simulink model "parcheggioAssistito_Simu"  (R2023a)
settings: Solver=VariableStepAuto  StartTime=0.0  StopTime=30.0  RelTol=1e-3
undefined symbols (not defined in the file or in its folder): ZigBee
libraries: truetime x12, fuzblock x1
settings Model: Creator=elisa  LastModifiedBy=elisa

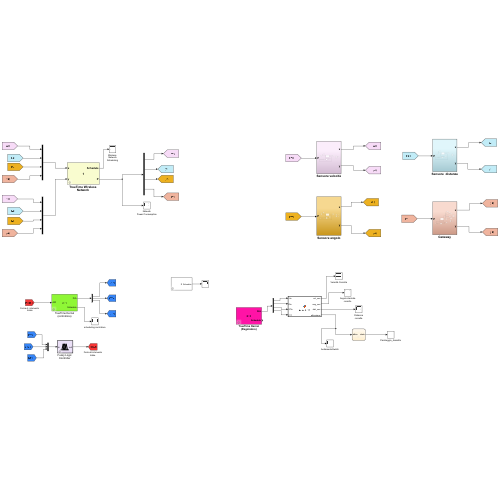
[thumbnail: Simulink's stored preview of the top-level diagram]
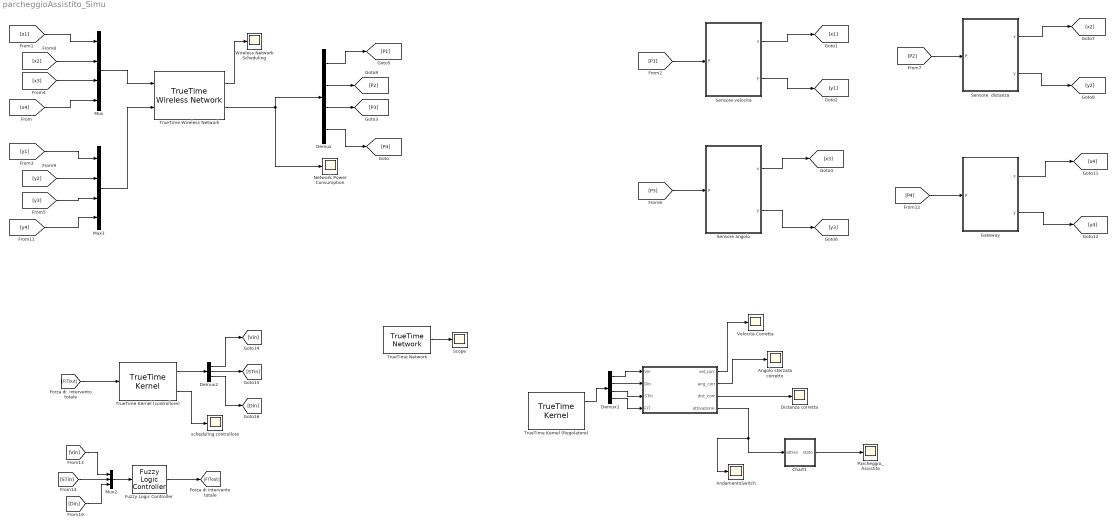
== system parcheggioAssistito_Simu ==
  " " : MATLAB Function  TreatAsAtomicUnit=on
  AndamentoSwitch : Scope
  Angolo sterzata corretto : Scope
  Chart1 : Stateflow chart  TreatAsAtomicUnit=on
  Demux : Demux
  Demux1 : Demux
  Demux2 : Demux  Outputs=3
  Distanza corretta : Scope
  "Fuzzy Logic Controller " : fuzblock/Fuzzy Logic  Controller  FIS='parcheggioAssistito.fis'  OutputSampleNumber=101  DataType=double  FuzzifiedInputs=off  RuleFiringStrengths=off  RuleOutputs=off  AggregatedOutputs=off  SimulateUsing=Interpreted execution  OutOfRangeInputValueMessage=warning  NoRuleFiredMessage=warning  EmptyOutputFuzzySetMessage=warning
  Gateway : Subsystem
  Mux : Mux
  Mux1 : Mux
  Mux2 : Mux  Inputs=3
  Network Power Consumption : Scope
  Parcheggio_Assistito : Scope
  Scope : Scope
  Sensore  distanza : Subsystem
  Sensore angolo : Subsystem
  Sensore velocità : Subsystem
  TrueTime Kernel (Regolatore) : truetime/TrueTime Kernel  sfun=regolatore_init  args=[]  ninputsoutputs=[0 4]  ntriggers=0  trigtype=falling  nwnodenbr=[2 3]  clockoffsetdrift=[0 0]  schedoutput=on  battery=off  poweroutput=off  label=2: 3
  TrueTime Kernel (controllore) : truetime/TrueTime Kernel  sfun=controllore_init  args=[]  ninputsoutputs=[1 3]  ntriggers=0  trigtype=falling  nwnodenbr=[2 1]  clockoffsetdrift=[0 0]  schedoutput=on  battery=off  poweroutput=off  label=2: 1
  TrueTime Network : truetime/TrueTime Network  nwtype=CSMA/CD (Ethernet)  nwnbr=2  nnodes=3  rate=10000000  minsize=512  lossprob=0  seed=0  bandwidths=[0.5 0.5]  slotsize=512  schedule=[1 1 2]  memsize=80000  buftype=Common buffer  overflow=Retransmit  dynSchedule=0  miniSlotSize=0  NIT=0  QSortMode=FIFO  sync=0  irtSchedule=0  nrtLength=0  nodeGraph=0  scheduleoutput=on
  "TrueTime Wireless Network " : truetime/TrueTime Wireless  Network  nwtype=802.15.4 (ZigBee)  nwnbr=1  nnodes=4  rate=800000  minsize=272  transpower=20  threshold=-48  use_pathloss_function=default  pathloss=3.5  acktimeout=0.00004  retrylimit=5  error_threshold=0.03  lossprob=0  seed=0  scheduleoutput=on  poweroutput=on
  Velocità Corretta : Scope
  Wireless Network Scheduling : Scope
  "scheduling controllore " : Scope
  wires:
  Sensore velocità/1(x) -> [x1]
  Sensore velocità/2(y) -> [y1]
  [P1] -> Sensore velocità/1(P)
  Sensore  distanza/1(x) -> [x2]
  Sensore  distanza/2(y) -> [y2]
  [P2] -> Sensore  distanza/1(P)
  [x1] -> Mux/1
  Demux/1 -> [P1]
  [y1] -> Mux1/1
  Mux/1 -> "TrueTime Wireless Network "/1
  "TrueTime Wireless Network "/2 -> Network Power Consumption/1, Demux/1
  "TrueTime Wireless Network "/1 -> Wireless Network Scheduling/1
  Mux1/1 -> "TrueTime Wireless Network "/2
  Demux/2 -> [P2]
  [x2] -> Mux/2
  [y2] -> Mux1/2
  [x3] -> Mux/3
  [y3] -> Mux1/3
  Demux/3 -> [P3]
  Sensore angolo/1(x) -> [x3]
  Sensore angolo/2(y) -> [y3]
  Demux/4 -> [P4]
  [y4] -> Mux1/4
  [x4] -> Mux/4
  [P3] -> Sensore angolo/1(P)
  Gateway/2(y) -> [y4]
  [P4] -> Gateway/1(P)
  Gateway/1(x) -> [x4]
  TrueTime Network/1 -> Scope/1
  [Vin] -> Mux2/1
  "Fuzzy Logic Controller "/1 -> [FITout]
  TrueTime Kernel (controllore)/1 -> Demux2/1
  [Din] -> Mux2/3
  Mux2/1 -> "Fuzzy Logic Controller "/1
  TrueTime Kernel (controllore)/2 -> "scheduling controllore "/1
  Demux2/1 -> [Vin]
  [FITout] -> TrueTime Kernel (controllore)/1
  Demux2/3 -> [Din]
  Demux2/2 -> [STin]
  [STin] -> Mux2/2
  " "/1(vel_corr) -> Velocità Corretta/1
  TrueTime Kernel (Regolatore)/1 -> Demux1/1
  " "/2(ang_corr) -> Angolo sterzata corretto/1
  " "/3(dist_corr) -> Distanza corretta/1
  Demux1/1 -> " "/1(Vin)
  Demux1/4 -> " "/4(FIT)
  Demux1/2 -> " "/2(Din)
  Demux1/3 -> " "/3(STin)
  " "/4(attivazione) -> Chart1/1(attiva), AndamentoSwitch/1
  Chart1/1(stato) -> Parcheggio_Assistito/1

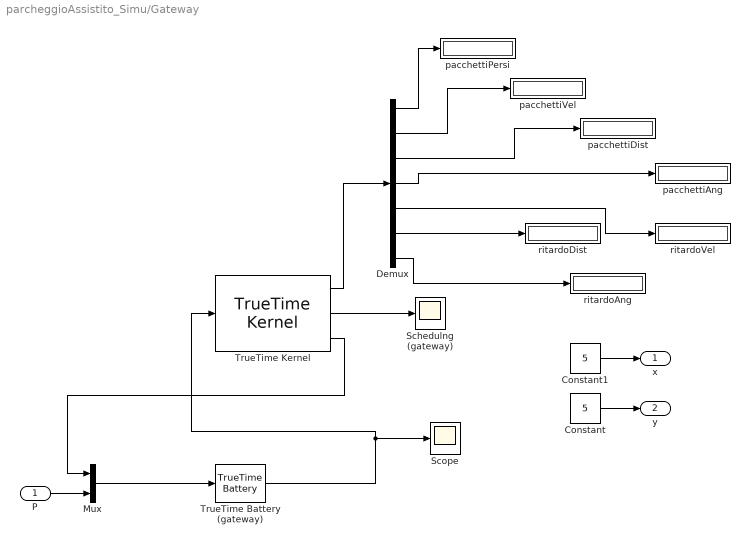
== system parcheggioAssistito_Simu/Gateway ==
  P : Inport
  Constant : Constant  Value=5
  Constant1 : Constant  Value=5
  Demux : Demux  Outputs=7
  Mux : Mux  Inputs=2
  Schedulng (gateway) : Scope
  Scope : Scope
  TrueTime Battery (gateway) : truetime/TrueTime Battery  energy=1
  TrueTime Kernel : truetime/TrueTime Kernel  sfun=gateway_init  args=[]  ninputsoutputs=[0 7]  ntriggers=0  trigtype=falling  nwnodenbr=[1 4; 2 2]  clockoffsetdrift=[0 0]  schedoutput=on  battery=on  poweroutput=on  label=1: 4\n2: 2
  pacchettiAng : Display
  pacchettiDist : Display
  pacchettiPersi : Display
  pacchettiVel : Display
  ritardoAng : Display
  ritardoDist : Display
  ritardoVel : Display
  x : Outport
  y : Outport  Port=2
  wires:
  TrueTime Kernel/3 -> Mux/1
  TrueTime Kernel/2 -> Schedulng (gateway)/1
  Mux/1 -> TrueTime Battery (gateway)/1
  Constant1/1 -> x/1
  P/1 -> Mux/2
  TrueTime Battery (gateway)/1 -> TrueTime Kernel/1, Scope/1
  Constant/1 -> y/1
  TrueTime Kernel/1 -> Demux/1
  Demux/1 -> pacchettiPersi/1
  Demux/2 -> pacchettiVel/1
  Demux/3 -> pacchettiDist/1
  Demux/4 -> pacchettiAng/1
  Demux/5 -> ritardoVel/1
  Demux/6 -> ritardoDist/1
  Demux/7 -> ritardoAng/1

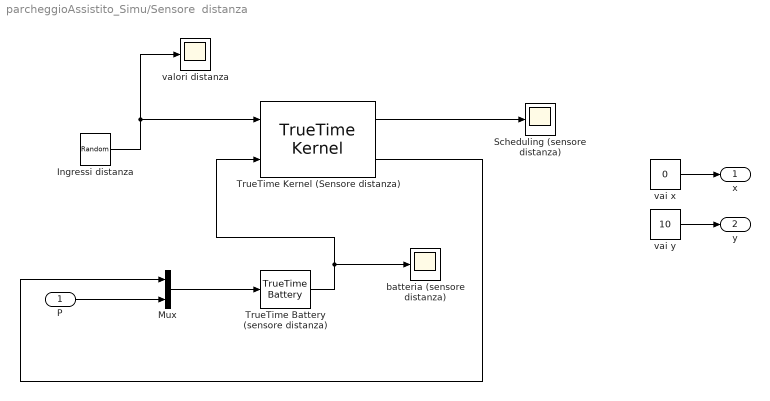
== system parcheggioAssistito_Simu/Sensore  distanza ==
  P : Inport
  Ingressi distanza : UniformRandomNumber  Minimum=0  Maximum=200  SampleTime=0.1
  Mux : Mux  Inputs=2
  Scheduling (sensore distanza) : Scope
  TrueTime Battery (sensore distanza) : truetime/TrueTime Battery  energy=3
  TrueTime Kernel (Sensore distanza) : truetime/TrueTime Kernel  sfun=sensore_distanza_init  args=[]  ninputsoutputs=[1 0]  ntriggers=0  trigtype=falling  nwnodenbr=[1 2]  clockoffsetdrift=[0 0]  schedoutput=on  battery=on  poweroutput=on  label=1: 2
  batteria (sensore distanza) : Scope
  vai x : Constant  Value=0
  vai y : Constant  Value=10
  valori distanza : Scope
  x : Outport
  y : Outport  Port=2
  wires:
  Mux/1 -> TrueTime Battery (sensore distanza)/1
  P/1 -> Mux/2
  TrueTime Kernel (Sensore distanza)/2 -> Mux/1
  TrueTime Battery (sensore distanza)/1 -> batteria (sensore distanza)/1, TrueTime Kernel (Sensore distanza)/2
  TrueTime Kernel (Sensore distanza)/1 -> Scheduling (sensore distanza)/1
  vai y/1 -> y/1
  vai x/1 -> x/1
  Ingressi distanza/1 -> valori distanza/1, TrueTime Kernel (Sensore distanza)/1

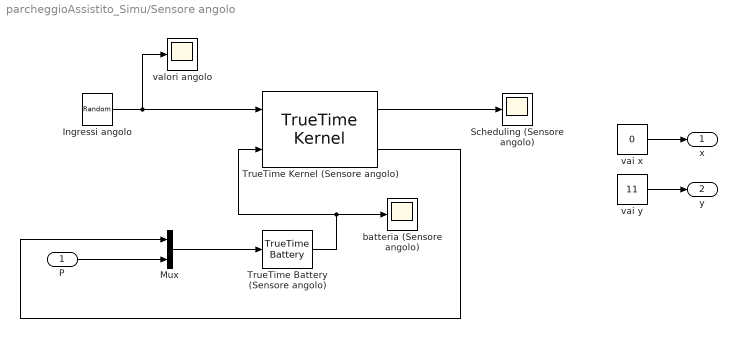
== system parcheggioAssistito_Simu/Sensore angolo ==
  P : Inport
  Ingressi angolo : UniformRandomNumber  Minimum=-30  Maximum=30  SampleTime=1
  Mux : Mux  Inputs=2
  Scheduling (Sensore angolo) : Scope
  TrueTime Battery (Sensore angolo) : truetime/TrueTime Battery  energy=3
  TrueTime Kernel (Sensore angolo) : truetime/TrueTime Kernel  sfun=sensore_angolo_init  args=[]  ninputsoutputs=[1 0]  ntriggers=0  trigtype=falling  nwnodenbr=[1 3]  clockoffsetdrift=[0 0]  schedoutput=on  battery=on  poweroutput=on  label=1: 3
  batteria (Sensore angolo) : Scope
  vai x : Constant  Value=0
  vai y : Constant  Value=11
  valori angolo : Scope
  x : Outport
  y : Outport  Port=2
  wires:
  Ingressi angolo/1 -> valori angolo/1, TrueTime Kernel (Sensore angolo)/1
  TrueTime Kernel (Sensore angolo)/1 -> Scheduling (Sensore angolo)/1
  vai x/1 -> x/1
  vai y/1 -> y/1
  P/1 -> Mux/2
  Mux/1 -> TrueTime Battery (Sensore angolo)/1
  TrueTime Battery (Sensore angolo)/1 -> batteria (Sensore angolo)/1, TrueTime Kernel (Sensore angolo)/2
  TrueTime Kernel (Sensore angolo)/2 -> Mux/1

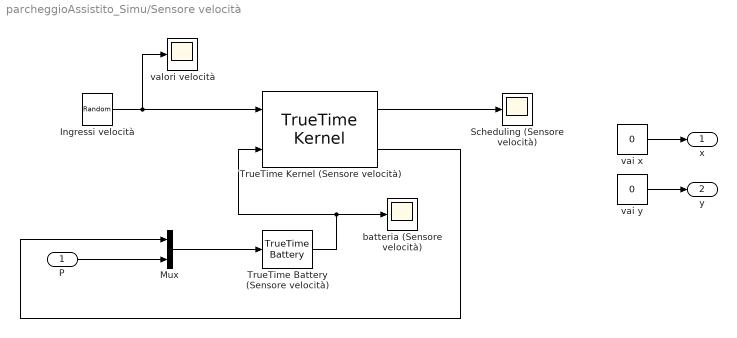
== system parcheggioAssistito_Simu/Sensore velocità ==
  P : Inport
  Ingressi velocità : UniformRandomNumber  Minimum=0  Maximum=20  SampleTime=1
  Mux : Mux  Inputs=2
  Scheduling (Sensore velocità) : Scope
  TrueTime Battery (Sensore velocità) : truetime/TrueTime Battery  energy=3
  TrueTime Kernel (Sensore velocità) : truetime/TrueTime Kernel  sfun=sensore_velocita_init  args=[]  ninputsoutputs=[1 0]  ntriggers=0  trigtype=falling  nwnodenbr=[1 1]  clockoffsetdrift=[0 0]  schedoutput=on  battery=on  poweroutput=on  label=1: 1
  batteria (Sensore velocità) : Scope
  vai x : Constant  Value=0
  vai y : Constant  Value=0
  valori velocità : Scope
  x : Outport
  y : Outport  Port=2
  wires:
  Mux/1 -> TrueTime Battery (Sensore velocità)/1
  P/1 -> Mux/2
  TrueTime Kernel (Sensore velocità)/2 -> Mux/1
  TrueTime Battery (Sensore velocità)/1 -> batteria (Sensore velocità)/1, TrueTime Kernel (Sensore velocità)/2
  TrueTime Kernel (Sensore velocità)/1 -> Scheduling (Sensore velocità)/1
  vai y/1 -> y/1
  vai x/1 -> x/1
  Ingressi velocità/1 -> valori velocità/1, TrueTime Kernel (Sensore velocità)/1

== stateflow chart parcheggioAssistito_Simu/Chart1 ==
  state OnOff
    state dispositivo_attivato
      switchP= 1;
    state Idle
      entry:
      stato = 0;
    state parcheggio_in_corso
      stato = 1;
      switchP = 0;
    Idle -> dispositivo_attivato : [attiva == 1]
    (default) -> Idle
    dispositivo_attivato -> parcheggio_in_corso : [switchP==1 &&attiva==1]
    parcheggio_in_corso -> Idle : [after(10,sec)]
  data: attiva input double; stato output uint8; switchP local uint8

== matlab function parcheggioAssistito_Simu/  ==
  data: Vin input; Din input; STin input; FIT input; vel_corr output; ang_corr output; dist_corr output; attivazione output
function [vel_corr, ang_corr, dist_corr, attivazione] = gestoreFIT(Vin, Din, STin, FIT)
    
    attivazione = 0; % parcheggio assistito non attivo
    
    % Target ideali
    target_vel  = 6;     % m/s o unità arbitrarie
    target_dist = 135;   % cm
    target_ang  = 0;     % sterzata ideale (dritta)

    % Calcolo fattore di correzione non lineare (tra 0 e 1)
    k = 1 - exp(-5 * FIT);  % cresce più dolcemente

    % Pesi sulle grandezze (priorità: velocità > distanza > angolo)
    w_vel  = 0.7;
    w_dist = 0.6;
    w_ang  = 0.5;


    % Se FIT è molto basso, lascia invariato
    if FIT < 0.4
        vel_corr  = Vin;
        dist_corr = Din;
        ang_corr  = STin;
        
    else

    % Applica correzione verso i target ideali
    attivazione = 1; % parcheggio assistito attivo
    vel_corr  = Vin  + (target_vel  - Vin)  * k * w_vel;
    dist_corr = Din  + (target_dist - Din) * k * w_dist;
    ang_corr  = STin + (target_ang  - STin) * k * w_ang;

    end
end
